simulink model "Perfect_Lineaer"  (R2017a)
settings: Solver=VariableStepAuto  StartTime=0.0  StopTime=17  FixedStep=0.01  RelTol=1e-3
values from neighbouring files (symbols this model uses):
  A = [-4.65E-06	0.0001701	-0.0002836	0	0	0	-2.56E-06	-7.97E-06	3.61E-06 ... (first row only)    [surfaces_setup_test.m]
  A0 = [-4.65E-06	0.0001701	-0.0002836	0	0	0	0	-1.43	0 ... (first row only)    [surfaces_setup_test.m]
  a0_s2345 = [0;0;0.05;0.05]    [HW5_4_surfaces.m]    (also in TEST_aerosetup.m; surfaces_setup_test.m)
  A_2345 = c_2345.*b_2345    [HW5_4_surfaces.m]    (also in TEST_aerosetup.m; surfaces_setup_test.m)
  Aileron_left = 0    [HW5_4_surfaces.m]    (also in TEST_aerosetup.m; surfaces_setup_test.m)
  Aileron_right = 0    [HW5_4_surfaces.m]    (also in TEST_aerosetup.m; surfaces_setup_test.m)
  B = [-7.98E-09	7.83E-09	1.68E-09	2.75E-10 ... (first row only)    [surfaces_setup_test.m]
  B0 = [-6.2	6.2	0	0.45 ... (first row only)    [surfaces_setup_test.m]
  c_2345 = [0.075;0.08;0.1;0.1]    [HW5_4_surfaces.m]    (also in TEST_aerosetup.m; surfaces_setup_test.m)
  CD0_s2345 = [0.01;0.01;0.01;0.01]    [HW5_4_surfaces.m]    (also in TEST_aerosetup.m; surfaces_setup_test.m)
  CDa_s2345 = [1;1;1;1]    [HW5_4_surfaces.m]    (also in TEST_aerosetup.m; surfaces_setup_test.m)
  CL0_2345 = [0;0; 0.05; 0.05]    [HW5_4_surfaces.m]    (also in TEST_aerosetup.m; surfaces_setup_test.m)
  CLa = 2*pi*(r./(2+r))    [HW5_4_surfaces.m]    (also in TEST_aerosetup.m; surfaces_setup_test.m)
  CM0_s2345 = [0;0;-0.05;-0.05]    [HW5_4_surfaces.m]    (also in TEST_aerosetup.m; surfaces_setup_test.m)
  CMa_s2345 = [0; 0; 0; 0]    [HW5_4_surfaces.m]    (also in TEST_aerosetup.m; surfaces_setup_test.m)
  e_s2345 = [0.8;0.8;0.9;0.9]    [HW5_4_surfaces.m]    (also in TEST_aerosetup.m; surfaces_setup_test.m)
  elevator = 0    [HW5_4_surfaces.m]    (also in TEST_aerosetup.m; surfaces_setup_test.m)
  Fext_N = -g_EN * m    [HW5_4_surfaces.m]    (also in TEST_aerosetup.m = [10 10 10]; surfaces_setup_test.m)
  g_EN = [0; 0; 9.81]    [HW5_4_surfaces.m]    (also in TEST_aerosetup.m = [0; 0; 9.8]; surfaces_setup_test.m)
  i_s2345 = [0; 0; 0.05; 0.05;]    [HW5_4_surfaces.m]    (also in TEST_aerosetup.m; surfaces_setup_test.m)
  J_cgp = ones(3)    [surfaces_setup_test.m]
  M_total = sum(MnG(:,1))/1000    [HW5_4_surfaces.m]    (also in TEST_aerosetup.m; surfaces_setup_test.m = sum(MnG1(:,1))/1000)
  Mext_B = [0; 0; 0]    [HW5_4_surfaces.m]    (also in TEST_aerosetup.m = [1; 1; 1]; surfaces_setup_test.m)
  p_E_BE_ini = p_E_BE_ini_deg .* [deg2rad; deg2rad; 1]    [HW5_4_surfaces.m]    (also in TEST_aerosetup.m; surfaces_setup_test.m)
  r = b_2345./c_2345    [HW5_4_surfaces.m]    (also in TEST_aerosetup.m; surfaces_setup_test.m)
  Rearth = 6371000    [HW5_4_surfaces.m]    (also in TEST_aerosetup.m; surfaces_setup_test.m)
  rudder = 0    [HW5_4_surfaces.m]    (also in TEST_aerosetup.m; surfaces_setup_test.m)
  Theta_ini = Theta_ini_deg * deg2rad    [HW5_4_surfaces.m]    (also in TEST_aerosetup.m; surfaces_setup_test.m)
  U0 = [Aileron_right;Aileron_left;elevator;rudder]    [surfaces_setup_test.m]
  v_N_AE = [0;0;0]    [HW5_4_surfaces.m]    (also in TEST_aerosetup.m; surfaces_setup_test.m)
  Vbbe_int = [10; 0; 0]    [HW5_4_surfaces.m]    (also in TEST_aerosetup.m; surfaces_setup_test.m = [5; 0; 0])
  w_B_BE_ini = [1e0; 1e-2; 1e-2]    [HW5_4_surfaces.m]    (also in TEST_aerosetup.m; surfaces_setup_test.m)
  X0 = [w_B_BE_ini;Theta_ini;Vbbe_int]    [surfaces_setup_test.m]
  xyz_s = [[-0.76 0 0.16];[-0.76 0 -0.09];[-0.23 0.44 0];[-0.23 -0.44 0];]    [HW5_4_surfaces.m]    (also in TEST_aerosetup.m; surfaces_setup_test.m)
undefined symbols (not defined in the file or in its folder): Discrete, Earth, K, Time, WGS84
libraries: simulink x83, aerolibfltsims x5, dspsrcs4 x4, simulink_extras x4, dspinverses x3, vrlib x2, sharedtransform x1, aerolibtransform2 x1, aerolibutil x1, sharedutil x1, ctrlSharedLib x1
(part 7 of 8)

== system Perfect_Lineaer/Command size/Subsystem3/selector ==
  note: Outer loop
  In1 : Inport
  Demux : Demux  Outputs=9
  Demux1 : Demux  Outputs=3
  MATLAB Function : MATLAB Function  TreatAsAtomicUnit=on
  Mux : Mux  Inputs=8
  Mux1 : Mux  Inputs=3
  Scope : Scope
  Terminator : Terminator
  Terminator1 : Terminator
  Terminator2 : Terminator
  Out1 : Outport
  Out2 : Outport  Port=2
  wires:
  Mux1/1 -> Scope/1
  Demux/9 -> Mux/8
  Demux/8 -> Out1/1
  Mux/1 -> Terminator/1
  Demux/7 -> Mux/7
  Demux/6 -> Mux/6, Mux1/3
  Demux/4 -> MATLAB Function/1(phi), Mux/4, Mux1/1
  In1/1 -> Demux/1
  Demux/2 -> MATLAB Function/5(R), Mux/2
  Demux/3 -> Mux/3
  Demux/1 -> MATLAB Function/4(Q), MATLAB Function/3(P), Mux/1
  Demux/5 -> MATLAB Function/2(theta), Mux/5, Mux1/2
  MATLAB Function/1(euler_dot) -> Demux1/1
  Demux1/2 -> Out2/1
  Demux1/1 -> Terminator1/1
  Demux1/3 -> Terminator2/1

== system Perfect_Lineaer/Command size/Subsystem4/selector ==
  note: Outer loop
  In1 : Inport
  Demux : Demux  Outputs=9
  Demux1 : Demux  Outputs=3
  MATLAB Function : MATLAB Function  TreatAsAtomicUnit=on
  Mux : Mux  Inputs=8
  Mux1 : Mux  Inputs=3
  Scope : Scope
  Terminator : Terminator
  Terminator1 : Terminator
  Terminator2 : Terminator
  Out1 : Outport
  Out2 : Outport  Port=2
  wires:
  Demux1/2 -> Terminator1/1
  Demux/7 -> Mux/7
  Demux/3 -> Mux/3
  Mux/1 -> Terminator/1
  Demux/2 -> MATLAB Function/5(R), Mux/2
  In1/1 -> Demux/1
  Demux/5 -> MATLAB Function/2(theta), Mux/5, Mux1/2
  Demux/9 -> Mux/8
  Demux/6 -> Mux/6, Mux1/3
  Demux1/3 -> Terminator2/1
  MATLAB Function/1(euler_dot) -> Demux1/1
  Mux1/1 -> Scope/1
  Demux/4 -> MATLAB Function/1(phi), Mux/4, Mux1/1
  Demux/1 -> MATLAB Function/4(Q), MATLAB Function/3(P), Mux/1
  Demux1/1 -> Out2/1
  Demux/8 -> Out1/1

== system Perfect_Lineaer/Command size/Subsystem9/selector ==
  note: Outer loop
  In1 : Inport
  Demux : Demux  Outputs=9
  Demux1 : Demux  Outputs=3
  MATLAB Function : MATLAB Function  TreatAsAtomicUnit=on
  Mux : Mux  Inputs=8
  Mux1 : Mux  Inputs=3
  Scope : Scope
  Terminator : Terminator
  Terminator1 : Terminator
  Terminator2 : Terminator
  Out1 : Outport
  Out2 : Outport  Port=2
  wires:
  Demux1/2 -> Terminator1/1
  Demux/7 -> Mux/7
  Demux/3 -> Mux/3
  Mux/1 -> Terminator/1
  Demux/2 -> MATLAB Function/5(R), Mux/2
  In1/1 -> Demux/1
  Demux/5 -> MATLAB Function/2(theta), Mux/5, Mux1/2
  Demux/9 -> Mux/8
  Demux/6 -> Mux/6, Mux1/3
  Demux1/3 -> Terminator2/1
  MATLAB Function/1(euler_dot) -> Demux1/1
  Mux1/1 -> Scope/1
  Demux/4 -> MATLAB Function/1(phi), Mux/4, Mux1/1
  Demux/1 -> MATLAB Function/4(Q), MATLAB Function/3(P), Mux/1
  Demux1/1 -> Out2/1
  Demux/8 -> Out1/1

== system Perfect_Lineaer/Decoupled/Subsystem/selector ==
  note: Outer loop
  In1 : Inport
  Demux : Demux  Outputs=9
  Demux1 : Demux  Outputs=3
  MATLAB Function : MATLAB Function  TreatAsAtomicUnit=on
  Mux : Mux  Inputs=8
  Mux1 : Mux  Inputs=3
  Scope : Scope
  Terminator : Terminator
  Terminator1 : Terminator
  Terminator2 : Terminator
  Out1 : Outport
  Out2 : Outport  Port=2
  wires:
  MATLAB Function/1(euler_dot) -> Demux1/1
  Demux1/1 -> Terminator1/1
  In1/1 -> Demux/1
  Demux/9 -> Mux/8
  Demux/5 -> MATLAB Function/2(theta), Mux/5, Mux1/2
  Demux/2 -> MATLAB Function/5(R), Mux/2
  Demux/6 -> Mux/6, Mux1/3
  Demux/1 -> MATLAB Function/4(Q), MATLAB Function/3(P), Mux/1
  Demux/3 -> Mux/3
  Mux/1 -> Terminator/1
  Demux/7 -> Mux/7
  Demux/4 -> MATLAB Function/1(phi), Mux/4, Mux1/1
  Demux/8 -> Out1/1
  Mux1/1 -> Scope/1
  Demux1/3 -> Out2/1
  Demux1/2 -> Terminator2/1

== system Perfect_Lineaer/Decoupled/Subsystem1/selector ==
  note: Outer loop
  In1 : Inport
  Demux : Demux  Outputs=9
  Demux1 : Demux  Outputs=3
  MATLAB Function : MATLAB Function  TreatAsAtomicUnit=on
  Mux : Mux  Inputs=8
  Mux1 : Mux  Inputs=3
  Scope : Scope
  Terminator : Terminator
  Terminator1 : Terminator
  Terminator2 : Terminator
  Out1 : Outport
  Out2 : Outport  Port=2
  wires:
  Mux1/1 -> Scope/1
  Demux/9 -> Mux/8
  Demux/8 -> Out1/1
  Mux/1 -> Terminator/1
  Demux/7 -> Mux/7
  Demux/6 -> Mux/6, Mux1/3
  Demux/4 -> MATLAB Function/1(phi), Mux/4, Mux1/1
  In1/1 -> Demux/1
  Demux/2 -> MATLAB Function/5(R), Mux/2
  Demux/3 -> Mux/3
  Demux/1 -> MATLAB Function/4(Q), MATLAB Function/3(P), Mux/1
  Demux/5 -> MATLAB Function/2(theta), Mux/5, Mux1/2
  MATLAB Function/1(euler_dot) -> Demux1/1
  Demux1/2 -> Out2/1
  Demux1/1 -> Terminator1/1
  Demux1/3 -> Terminator2/1

== system Perfect_Lineaer/Decoupled/Subsystem5/selector ==
  note: Outer loop
  In1 : Inport
  Demux : Demux  Outputs=9
  Demux1 : Demux  Outputs=3
  MATLAB Function : MATLAB Function  TreatAsAtomicUnit=on
  Mux : Mux  Inputs=8
  Mux1 : Mux  Inputs=3
  Scope : Scope
  Terminator : Terminator
  Terminator1 : Terminator
  Out1 : Outport
  Out2 : Outport  Port=2
  Out3 : Outport  Port=3
  wires:
  MATLAB Function/1(euler_dot) -> Demux1/1
  Demux1/1 -> Terminator1/1
  In1/1 -> Demux/1
  Demux/9 -> Mux/8
  Demux/5 -> MATLAB Function/2(theta), Mux/5, Mux1/2
  Demux/2 -> MATLAB Function/5(R), Mux/2
  Demux/6 -> Mux/6, Mux1/3
  Demux/1 -> MATLAB Function/4(Q), MATLAB Function/3(P), Mux/1
  Demux/3 -> Mux/3
  Mux/1 -> Terminator/1
  Demux/7 -> Mux/7
  Demux/4 -> MATLAB Function/1(phi), Mux/4, Mux1/1
  Demux1/2 -> Out2/1
  Demux/8 -> Out1/1
  Mux1/1 -> Scope/1
  Demux1/3 -> Out3/1

== system Perfect_Lineaer/Decoupled/Subsystem9/selector ==
  note: Outer loop
  In1 : Inport
  Demux : Demux  Outputs=9
  Demux1 : Demux  Outputs=3
  MATLAB Function : MATLAB Function  TreatAsAtomicUnit=on
  Mux : Mux  Inputs=8
  Mux1 : Mux  Inputs=3
  Scope : Scope
  Terminator : Terminator
  Terminator1 : Terminator
  Terminator2 : Terminator
  Out1 : Outport
  Out2 : Outport  Port=2
  wires:
  Demux1/2 -> Terminator1/1
  Demux/7 -> Mux/7
  Demux/3 -> Mux/3
  Mux/1 -> Terminator/1
  Demux/2 -> MATLAB Function/5(R), Mux/2
  In1/1 -> Demux/1
  Demux/5 -> MATLAB Function/2(theta), Mux/5, Mux1/2
  Demux/9 -> Mux/8
  Demux/6 -> Mux/6, Mux1/3
  Demux1/3 -> Terminator2/1
  MATLAB Function/1(euler_dot) -> Demux1/1
  Mux1/1 -> Scope/1
  Demux/4 -> MATLAB Function/1(phi), Mux/4, Mux1/1
  Demux/1 -> MATLAB Function/4(Q), MATLAB Function/3(P), Mux/1
  Demux1/1 -> Out2/1
  Demux/8 -> Out1/1

== system Perfect_Lineaer/Pilot command(STT)/Subsystem/selector ==
  note: Outer loop
  In1 : Inport
  Demux : Demux  Outputs=9
  Demux1 : Demux  Outputs=3
  MATLAB Function : MATLAB Function  TreatAsAtomicUnit=on
  Mux : Mux  Inputs=8
  Mux1 : Mux  Inputs=3
  Scope : Scope
  Terminator : Terminator
  Terminator1 : Terminator
  Terminator2 : Terminator
  Out1 : Outport
  Out2 : Outport  Port=2
  wires:
  MATLAB Function/1(euler_dot) -> Demux1/1
  Demux1/1 -> Terminator1/1
  In1/1 -> Demux/1
  Demux/9 -> Mux/8
  Demux/5 -> MATLAB Function/2(theta), Mux/5, Mux1/2
  Demux/2 -> MATLAB Function/5(R), Mux/2
  Demux/6 -> Mux/6, Mux1/3
  Demux/1 -> MATLAB Function/4(Q), MATLAB Function/3(P), Mux/1
  Demux/3 -> Mux/3
  Mux/1 -> Terminator/1
  Demux/7 -> Mux/7
  Demux/4 -> MATLAB Function/1(phi), Mux/4, Mux1/1
  Demux/8 -> Out1/1
  Mux1/1 -> Scope/1
  Demux1/3 -> Out2/1
  Demux1/2 -> Terminator2/1

== system Perfect_Lineaer/Pilot command(STT)/Subsystem1/selector ==
  note: Outer loop
  In1 : Inport
  Demux : Demux  Outputs=9
  Demux1 : Demux  Outputs=3
  MATLAB Function : MATLAB Function  TreatAsAtomicUnit=on
  Mux : Mux  Inputs=8
  Mux1 : Mux  Inputs=3
  Scope : Scope
  Terminator : Terminator
  Terminator1 : Terminator
  Terminator2 : Terminator
  Out1 : Outport
  Out2 : Outport  Port=2
  wires:
  Mux1/1 -> Scope/1
  Demux/9 -> Mux/8
  Demux/8 -> Out1/1
  Mux/1 -> Terminator/1
  Demux/7 -> Mux/7
  Demux/6 -> Mux/6, Mux1/3
  Demux/4 -> MATLAB Function/1(phi), Mux/4, Mux1/1
  In1/1 -> Demux/1
  Demux/2 -> MATLAB Function/5(R), Mux/2
  Demux/3 -> Mux/3
  Demux/1 -> MATLAB Function/4(Q), MATLAB Function/3(P), Mux/1
  Demux/5 -> MATLAB Function/2(theta), Mux/5, Mux1/2
  MATLAB Function/1(euler_dot) -> Demux1/1
  Demux1/2 -> Out2/1
  Demux1/1 -> Terminator1/1
  Demux1/3 -> Terminator2/1

== system Perfect_Lineaer/Pilot command(STT)/Subsystem5/selector ==
  note: Outer loop
  In1 : Inport
  Demux : Demux  Outputs=9
  Demux1 : Demux  Outputs=3
  MATLAB Function : MATLAB Function  TreatAsAtomicUnit=on
  Mux : Mux  Inputs=8
  Mux1 : Mux  Inputs=3
  Scope : Scope
  Terminator : Terminator
  Terminator1 : Terminator
  Out1 : Outport
  Out2 : Outport  Port=2
  Out3 : Outport  Port=3
  wires:
  MATLAB Function/1(euler_dot) -> Demux1/1
  Demux1/1 -> Terminator1/1
  In1/1 -> Demux/1
  Demux/9 -> Mux/8
  Demux/5 -> MATLAB Function/2(theta), Mux/5, Mux1/2
  Demux/2 -> MATLAB Function/5(R), Mux/2
  Demux/6 -> Mux/6, Mux1/3
  Demux/1 -> MATLAB Function/4(Q), MATLAB Function/3(P), Mux/1
  Demux/3 -> Mux/3
  Mux/1 -> Terminator/1
  Demux/7 -> Mux/7
  Demux/4 -> MATLAB Function/1(phi), Mux/4, Mux1/1
  Demux1/2 -> Out2/1
  Demux/8 -> Out1/1
  Mux1/1 -> Scope/1
  Demux1/3 -> Out3/1

== system Perfect_Lineaer/Really skid to turn/Subsystem5/selector ==
  note: Outer loop
  In1 : Inport
  Demux : Demux  Outputs=9
  Demux1 : Demux  Outputs=3
  MATLAB Function : MATLAB Function  TreatAsAtomicUnit=on
  Mux : Mux  Inputs=8
  Mux1 : Mux  Inputs=3
  Scope : Scope
  Terminator : Terminator
  Terminator1 : Terminator
  Out1 : Outport
  Out2 : Outport  Port=2
  Out3 : Outport  Port=3
  wires:
  MATLAB Function/1(euler_dot) -> Demux1/1
  Demux1/1 -> Terminator1/1
  In1/1 -> Demux/1
  Demux/9 -> Mux/8
  Demux/5 -> MATLAB Function/2(theta), Mux/5, Mux1/2
  Demux/2 -> MATLAB Function/5(R), Mux/2
  Demux/6 -> Mux/6, Mux1/3
  Demux/1 -> MATLAB Function/4(Q), MATLAB Function/3(P), Mux/1
  Demux/3 -> Mux/3
  Mux/1 -> Terminator/1
  Demux/7 -> Mux/7
  Demux/4 -> MATLAB Function/1(phi), Mux/4, Mux1/1
  Demux1/2 -> Out2/1
  Demux/8 -> Out1/1
  Mux1/1 -> Scope/1
  Demux1/3 -> Out3/1

== system Perfect_Lineaer/Really skid to turn/Subsystem8/selector ==
  note: Outer loop
  In1 : Inport
  Demux : Demux  Outputs=9
  Demux1 : Demux  Outputs=3
  MATLAB Function : MATLAB Function  TreatAsAtomicUnit=on
  Mux : Mux  Inputs=8
  Mux1 : Mux  Inputs=3
  Scope : Scope
  Terminator : Terminator
  Terminator1 : Terminator
  Terminator2 : Terminator
  Out1 : Outport
  Out2 : Outport  Port=2
  wires:
  Demux1/2 -> Terminator1/1
  Demux/7 -> Mux/7
  Demux/3 -> Mux/3
  Mux/1 -> Terminator/1
  Demux/2 -> MATLAB Function/5(R), Mux/2
  In1/1 -> Demux/1
  Demux/5 -> MATLAB Function/2(theta), Mux/5, Mux1/2
  Demux/9 -> Mux/8
  Demux/6 -> Mux/6, Mux1/3
  Demux1/3 -> Terminator2/1
  MATLAB Function/1(euler_dot) -> Demux1/1
  Mux1/1 -> Scope/1
  Demux/4 -> MATLAB Function/1(phi), Mux/4, Mux1/1
  Demux/1 -> MATLAB Function/4(Q), MATLAB Function/3(P), Mux/1
  Demux1/1 -> Out2/1
  Demux/8 -> Out1/1

== system Perfect_Lineaer/Really skid to turn/Subsystem9/selector ==
  note: Outer loop
  In1 : Inport
  Demux : Demux  Outputs=9
  Demux1 : Demux  Outputs=3
  MATLAB Function : MATLAB Function  TreatAsAtomicUnit=on
  Mux : Mux  Inputs=8
  Mux1 : Mux  Inputs=3
  Scope : Scope
  Terminator : Terminator
  Terminator1 : Terminator
  Terminator2 : Terminator
  Out1 : Outport
  Out2 : Outport  Port=2
  wires:
  Demux1/2 -> Terminator1/1
  Demux/7 -> Mux/7
  Demux/3 -> Mux/3
  Mux/1 -> Terminator/1
  Demux/2 -> MATLAB Function/5(R), Mux/2
  In1/1 -> Demux/1
  Demux/5 -> MATLAB Function/2(theta), Mux/5, Mux1/2
  Demux/9 -> Mux/8
  Demux/6 -> Mux/6, Mux1/3
  Demux1/3 -> Terminator2/1
  MATLAB Function/1(euler_dot) -> Demux1/1
  Mux1/1 -> Scope/1
  Demux/4 -> MATLAB Function/1(phi), Mux/4, Mux1/1
  Demux/1 -> MATLAB Function/4(Q), MATLAB Function/3(P), Mux/1
  Demux1/1 -> Out2/1
  Demux/8 -> Out1/1

== system Perfect_Lineaer/Skid to turn (Lateral Dynamics don't change!)/Subsystem/selector ==
  note: Outer loop
  In1 : Inport
  Demux : Demux  Outputs=9
  Mux : Mux  Inputs=8
  Mux1 : Mux  Inputs=3
  Scope : Scope
  Terminator : Terminator
  Out1 : Outport
  Out2 : Outport  Port=2
  wires:
  Demux/5 -> Mux1/2, Mux/5
  Demux/1 -> Mux/1
  Demux/3 -> Out2/1, Mux/3
  Demux/2 -> Mux/2
  In1/1 -> Demux/1
  Demux/4 -> Mux1/1, Mux/4
  Demux/6 -> Mux1/3, Mux/6
  Demux/7 -> Mux/7
  Mux/1 -> Terminator/1
  Demux/8 -> Out1/1
  Demux/9 -> Mux/8
  Mux1/1 -> Scope/1

== system Perfect_Lineaer/Skid to turn (Lateral Dynamics don't change!)/Subsystem1/selector ==
  note: Outer loop
  In1 : Inport
  Demux : Demux  Outputs=9
  Mux : Mux  Inputs=8
  Mux1 : Mux  Inputs=3
  Scope : Scope
  Terminator : Terminator
  Out1 : Outport
  Out2 : Outport  Port=2
  wires:
  Demux/5 -> Mux1/2, Mux/5
  Demux/1 -> Mux/1
  Demux/3 -> Mux/3
  Demux/2 -> Out2/1, Mux/2
  In1/1 -> Demux/1
  Demux/4 -> Mux1/1, Mux/4
  Demux/6 -> Mux1/3, Mux/6
  Demux/7 -> Mux/7
  Mux/1 -> Terminator/1
  Demux/8 -> Out1/1
  Demux/9 -> Mux/8
  Mux1/1 -> Scope/1

== system Perfect_Lineaer/Skid to turn (Lateral Dynamics don't change!)/Subsystem2/selector ==
  note: Outer loop
  In1 : Inport
  Demux : Demux  Outputs=9
  Mux : Mux  Inputs=8
  Mux1 : Mux  Inputs=3
  Scope : Scope
  Terminator : Terminator
  Out1 : Outport
  Out2 : Outport  Port=2
  wires:
  Demux/5 -> Mux1/2, Mux/5
  Demux/1 -> Mux/1
  Demux/3 -> Out2/1, Mux/3
  Demux/2 -> Mux/2
  In1/1 -> Demux/1
  Demux/4 -> Mux1/1, Mux/4
  Demux/6 -> Mux1/3, Mux/6
  Demux/7 -> Mux/7
  Mux/1 -> Terminator/1
  Demux/8 -> Out1/1
  Demux/9 -> Mux/8
  Mux1/1 -> Scope/1

== system Perfect_Lineaer/Skid to turn (Lateral Dynamics don't change!)/Subsystem3/selector ==
  note: Outer loop
  In1 : Inport
  Demux : Demux  Outputs=9
  Mux : Mux  Inputs=8
  Mux1 : Mux  Inputs=3
  Scope : Scope
  Terminator : Terminator
  Out1 : Outport
  Out2 : Outport  Port=2
  wires:
  Demux/5 -> Mux1/2, Mux/5
  Demux/1 -> Mux/1
  Demux/3 -> Out2/1, Mux/3
  Demux/2 -> Mux/2
  In1/1 -> Demux/1
  Demux/4 -> Mux1/1, Mux/4
  Demux/6 -> Mux1/3, Mux/6
  Demux/7 -> Mux/7
  Mux/1 -> Terminator/1
  Demux/8 -> Out1/1
  Demux/9 -> Mux/8
  Mux1/1 -> Scope/1

== system Perfect_Lineaer/Skid to turn (Lateral Dynamics don't change!)/Subsystem4/selector ==
  note: Outer loop
  In1 : Inport
  Demux : Demux  Outputs=9
  Mux : Mux  Inputs=8
  Mux1 : Mux  Inputs=3
  Scope : Scope
  Terminator : Terminator
  Out1 : Outport
  Out2 : Outport  Port=2
  wires:
  Demux/5 -> Mux1/2, Mux/5
  Demux/1 -> Mux/1
  Demux/3 -> Out2/1, Mux/3
  Demux/2 -> Mux/2
  In1/1 -> Demux/1
  Demux/4 -> Mux1/1, Mux/4
  Demux/6 -> Mux1/3, Mux/6
  Demux/7 -> Mux/7
  Mux/1 -> Terminator/1
  Demux/8 -> Out1/1
  Demux/9 -> Mux/8
  Mux1/1 -> Scope/1

== system Perfect_Lineaer/Skid to turn (Lateral Dynamics don't change!)/Subsystem5/selector ==
  note: Outer loop
  In1 : Inport
  Demux : Demux  Outputs=9
  Mux : Mux  Inputs=8
  Mux1 : Mux  Inputs=3
  Scope : Scope
  Terminator : Terminator
  Out1 : Outport
  yaw : Outport  Port=2
  pitch : Outport  Port=3
  wires:
  Demux/5 -> Mux1/2, Mux/5
  Demux/1 -> Mux/1
  Demux/3 -> yaw/1, Mux/3
  Demux/2 -> pitch/1, Mux/2
  In1/1 -> Demux/1
  Demux/4 -> Mux1/1, Mux/4
  Demux/6 -> Mux1/3, Mux/6
  Demux/7 -> Mux/7
  Mux/1 -> Terminator/1
  Demux/8 -> Out1/1
  Demux/9 -> Mux/8
  Mux1/1 -> Scope/1

== system Perfect_Lineaer/Skid to turn (Lateral Dynamics don't change!)/Subsystem6/selector ==
  note: Outer loop
  In1 : Inport
  Demux : Demux  Outputs=9
  Mux : Mux  Inputs=8
  Mux1 : Mux  Inputs=3
  Scope : Scope
  Terminator : Terminator
  Out1 : Outport
  Out2 : Outport  Port=2
  wires:
  Demux/5 -> Mux1/2, Mux/5
  Demux/1 -> Mux/1
  Demux/3 -> Out2/1, Mux/3
  Demux/2 -> Mux/2
  In1/1 -> Demux/1
  Demux/4 -> Mux1/1, Mux/4
  Demux/6 -> Mux1/3, Mux/6
  Demux/7 -> Mux/7
  Mux/1 -> Terminator/1
  Demux/8 -> Out1/1
  Demux/9 -> Mux/8
  Mux1/1 -> Scope/1

== system Perfect_Lineaer/Skid to turn (Lateral Dynamics don't change!)/Subsystem7/selector ==
  note: Outer loop
  In1 : Inport
  Demux : Demux  Outputs=9
  Mux : Mux  Inputs=8
  Mux1 : Mux  Inputs=3
  Scope : Scope
  Terminator : Terminator
  Out1 : Outport
  Out2 : Outport  Port=2
  wires:
  Demux/5 -> Mux1/2, Mux/5
  Demux/1 -> Out2/1, Mux/1
  Demux/3 -> Mux/3
  Demux/2 -> Mux/2
  In1/1 -> Demux/1
  Demux/4 -> Mux1/1, Mux/4
  Demux/6 -> Mux1/3, Mux/6
  Demux/7 -> Mux/7
  Mux/1 -> Terminator/1
  Demux/8 -> Out1/1
  Demux/9 -> Mux/8
  Mux1/1 -> Scope/1

== system Perfect_Lineaer/Skid to turn (Lateral Dynamics don't change!)/Subsystem8/selector ==
  note: Outer loop
  In1 : Inport
  Demux : Demux  Outputs=9
  Mux : Mux  Inputs=8
  Mux1 : Mux  Inputs=3
  Scope : Scope
  Terminator : Terminator
  Out1 : Outport
  Out2 : Outport  Port=2
  wires:
  Demux/5 -> Mux1/2, Mux/5
  Demux/1 -> Out2/1, Mux/1
  Demux/3 -> Mux/3
  Demux/2 -> Mux/2
  In1/1 -> Demux/1
  Demux/4 -> Mux1/1, Mux/4
  Demux/6 -> Mux1/3, Mux/6
  Demux/7 -> Mux/7
  Mux/1 -> Terminator/1
  Demux/8 -> Out1/1
  Demux/9 -> Mux/8
  Mux1/1 -> Scope/1

== system Perfect_Lineaer/Skid to turn (Lateral Dynamics don't change!)/Subsystem9/selector ==
  note: Outer loop
  In1 : Inport
  Demux : Demux  Outputs=9
  Mux : Mux  Inputs=8
  Mux1 : Mux  Inputs=3
  Scope : Scope
  Terminator : Terminator
  Out1 : Outport
  Out2 : Outport  Port=2
  wires:
  Demux/5 -> Mux1/2, Mux/5
  Demux/1 -> Out2/1, Mux/1
  Demux/3 -> Mux/3
  Demux/2 -> Mux/2
  In1/1 -> Demux/1
  Demux/4 -> Mux1/1, Mux/4
  Demux/6 -> Mux1/3, Mux/6
  Demux/7 -> Mux/7
  Mux/1 -> Terminator/1
  Demux/8 -> Out1/1
  Demux/9 -> Mux/8
  Mux1/1 -> Scope/1

== system Perfect_Lineaer/Skid to turn (Lateral Dynamics)1/Subsystem/selector ==
  note: Outer loop
  In1 : Inport
  Demux : Demux  Outputs=9
  Mux : Mux  Inputs=8
  Mux1 : Mux  Inputs=3
  Scope : Scope
  Terminator : Terminator
  Out1 : Outport
  Out2 : Outport  Port=2
  wires:
  Demux/5 -> Mux1/2, Mux/5
  Demux/1 -> Mux/1
  Demux/3 -> Out2/1, Mux/3
  Demux/2 -> Mux/2
  In1/1 -> Demux/1
  Demux/4 -> Mux1/1, Mux/4
  Demux/6 -> Mux1/3, Mux/6
  Demux/7 -> Mux/7
  Mux/1 -> Terminator/1
  Demux/8 -> Out1/1
  Demux/9 -> Mux/8
  Mux1/1 -> Scope/1

== system Perfect_Lineaer/Skid to turn (Lateral Dynamics)1/Subsystem1/selector ==
  note: Outer loop
  In1 : Inport
  Demux : Demux  Outputs=9
  Mux : Mux  Inputs=8
  Mux1 : Mux  Inputs=3
  Scope : Scope
  Terminator : Terminator
  Out1 : Outport
  Out2 : Outport  Port=2
  wires:
  Demux/5 -> Mux1/2, Mux/5
  Demux/1 -> Mux/1
  Demux/3 -> Mux/3
  Demux/2 -> Out2/1, Mux/2
  In1/1 -> Demux/1
  Demux/4 -> Mux1/1, Mux/4
  Demux/6 -> Mux1/3, Mux/6
  Demux/7 -> Mux/7
  Mux/1 -> Terminator/1
  Demux/8 -> Out1/1
  Demux/9 -> Mux/8
  Mux1/1 -> Scope/1

== system Perfect_Lineaer/Skid to turn (Lateral Dynamics)1/Subsystem2/selector ==
  note: Outer loop
  In1 : Inport
  Demux : Demux  Outputs=9
  Mux : Mux  Inputs=8
  Mux1 : Mux  Inputs=3
  Scope : Scope
  Terminator : Terminator
  Out1 : Outport
  Out2 : Outport  Port=2
  wires:
  Demux/5 -> Mux1/2, Mux/5
  Demux/1 -> Mux/1
  Demux/3 -> Out2/1, Mux/3
  Demux/2 -> Mux/2
  In1/1 -> Demux/1
  Demux/4 -> Mux1/1, Mux/4
  Demux/6 -> Mux1/3, Mux/6
  Demux/7 -> Mux/7
  Mux/1 -> Terminator/1
  Demux/8 -> Out1/1
  Demux/9 -> Mux/8
  Mux1/1 -> Scope/1

== system Perfect_Lineaer/Skid to turn (Lateral Dynamics)1/Subsystem3/selector ==
  note: Outer loop
  In1 : Inport
  Demux : Demux  Outputs=9
  Mux : Mux  Inputs=8
  Mux1 : Mux  Inputs=3
  Scope : Scope
  Terminator : Terminator
  Out1 : Outport
  Out2 : Outport  Port=2
  wires:
  Demux/5 -> Mux1/2, Mux/5
  Demux/1 -> Mux/1
  Demux/3 -> Out2/1, Mux/3
  Demux/2 -> Mux/2
  In1/1 -> Demux/1
  Demux/4 -> Mux1/1, Mux/4
  Demux/6 -> Mux1/3, Mux/6
  Demux/7 -> Mux/7
  Mux/1 -> Terminator/1
  Demux/8 -> Out1/1
  Demux/9 -> Mux/8
  Mux1/1 -> Scope/1

== system Perfect_Lineaer/Skid to turn (Lateral Dynamics)1/Subsystem4/selector ==
  note: Outer loop
  In1 : Inport
  Demux : Demux  Outputs=9
  Mux : Mux  Inputs=8
  Mux1 : Mux  Inputs=3
  Scope : Scope
  Terminator : Terminator
  Out1 : Outport
  Out2 : Outport  Port=2
  wires:
  Demux/5 -> Mux1/2, Mux/5
  Demux/1 -> Mux/1
  Demux/3 -> Out2/1, Mux/3
  Demux/2 -> Mux/2
  In1/1 -> Demux/1
  Demux/4 -> Mux1/1, Mux/4
  Demux/6 -> Mux1/3, Mux/6
  Demux/7 -> Mux/7
  Mux/1 -> Terminator/1
  Demux/8 -> Out1/1
  Demux/9 -> Mux/8
  Mux1/1 -> Scope/1

== system Perfect_Lineaer/Skid to turn (Lateral Dynamics)1/Subsystem5/selector ==
  note: Outer loop
  In1 : Inport
  Demux : Demux  Outputs=9
  Mux : Mux  Inputs=8
  Mux1 : Mux  Inputs=3
  Scope : Scope
  Terminator : Terminator
  Out1 : Outport
  yaw : Outport  Port=2
  pitch : Outport  Port=3
  wires:
  Demux/5 -> Mux1/2, Mux/5
  Demux/1 -> Mux/1
  Demux/3 -> yaw/1, Mux/3
  Demux/2 -> pitch/1, Mux/2
  In1/1 -> Demux/1
  Demux/4 -> Mux1/1, Mux/4
  Demux/6 -> Mux1/3, Mux/6
  Demux/7 -> Mux/7
  Mux/1 -> Terminator/1
  Demux/8 -> Out1/1
  Demux/9 -> Mux/8
  Mux1/1 -> Scope/1

== system Perfect_Lineaer/Skid to turn (Lateral Dynamics)1/Subsystem6/selector ==
  note: Outer loop
  In1 : Inport
  Demux : Demux  Outputs=9
  Mux : Mux  Inputs=8
  Mux1 : Mux  Inputs=3
  Scope : Scope
  Terminator : Terminator
  Out1 : Outport
  Out2 : Outport  Port=2
  wires:
  Demux/5 -> Mux1/2, Mux/5
  Demux/1 -> Mux/1
  Demux/3 -> Out2/1, Mux/3
  Demux/2 -> Mux/2
  In1/1 -> Demux/1
  Demux/4 -> Mux1/1, Mux/4
  Demux/6 -> Mux1/3, Mux/6
  Demux/7 -> Mux/7
  Mux/1 -> Terminator/1
  Demux/8 -> Out1/1
  Demux/9 -> Mux/8
  Mux1/1 -> Scope/1

== system Perfect_Lineaer/Skid to turn (Lateral Dynamics)1/Subsystem7/selector ==
  note: Outer loop
  In1 : Inport
  Demux : Demux  Outputs=9
  Mux : Mux  Inputs=8
  Mux1 : Mux  Inputs=3
  Scope : Scope
  Terminator : Terminator
  Out1 : Outport
  Out2 : Outport  Port=2
  wires:
  Demux/5 -> Mux1/2, Mux/5
  Demux/1 -> Out2/1, Mux/1
  Demux/3 -> Mux/3
  Demux/2 -> Mux/2
  In1/1 -> Demux/1
  Demux/4 -> Mux1/1, Mux/4
  Demux/6 -> Mux1/3, Mux/6
  Demux/7 -> Mux/7
  Mux/1 -> Terminator/1
  Demux/8 -> Out1/1
  Demux/9 -> Mux/8
  Mux1/1 -> Scope/1

== system Perfect_Lineaer/Skid to turn (Lateral Dynamics)1/Subsystem8/selector ==
  note: Outer loop
  In1 : Inport
  Demux : Demux  Outputs=9
  Mux : Mux  Inputs=8
  Mux1 : Mux  Inputs=3
  Scope : Scope
  Terminator : Terminator
  Out1 : Outport
  Out2 : Outport  Port=2
  wires:
  Demux/5 -> Mux1/2, Mux/5
  Demux/1 -> Out2/1, Mux/1
  Demux/3 -> Mux/3
  Demux/2 -> Mux/2
  In1/1 -> Demux/1
  Demux/4 -> Mux1/1, Mux/4
  Demux/6 -> Mux1/3, Mux/6
  Demux/7 -> Mux/7
  Mux/1 -> Terminator/1
  Demux/8 -> Out1/1
  Demux/9 -> Mux/8
  Mux1/1 -> Scope/1

== system Perfect_Lineaer/Skid to turn (Lateral Dynamics)1/Subsystem9/selector ==
  note: Outer loop
  In1 : Inport
  Demux : Demux  Outputs=9
  Mux : Mux  Inputs=8
  Mux1 : Mux  Inputs=3
  Scope : Scope
  Terminator : Terminator
  Out1 : Outport
  Out2 : Outport  Port=2
  wires:
  Demux/5 -> Mux1/2, Mux/5
  Demux/1 -> Out2/1, Mux/1
  Demux/3 -> Mux/3
  Demux/2 -> Mux/2
  In1/1 -> Demux/1
  Demux/4 -> Mux1/1, Mux/4
  Demux/6 -> Mux1/3, Mux/6
  Demux/7 -> Mux/7
  Mux/1 -> Terminator/1
  Demux/8 -> Out1/1
  Demux/9 -> Mux/8
  Mux1/1 -> Scope/1

== system Perfect_Lineaer/Skid to turn (Lateral Dynamics)2/Subsystem/selector ==
  note: Outer loop
  In1 : Inport
  Demux : Demux  Outputs=9
  Demux1 : Demux  Outputs=3
  MATLAB Function : MATLAB Function  TreatAsAtomicUnit=on
  Mux : Mux  Inputs=8
  Mux1 : Mux  Inputs=3
  Scope : Scope
  Terminator : Terminator
  Terminator1 : Terminator
  Terminator2 : Terminator
  Out1 : Outport
  Out2 : Outport  Port=2
  wires:
  MATLAB Function/1(euler_dot) -> Demux1/1
  Demux1/1 -> Terminator1/1
  In1/1 -> Demux/1
  Demux/9 -> Mux/8
  Demux/5 -> MATLAB Function/2(theta), Mux/5, Mux1/2
  Demux/2 -> MATLAB Function/5(R), Mux/2
  Demux/6 -> Mux/6, Mux1/3
  Demux/1 -> MATLAB Function/4(Q), MATLAB Function/3(P), Mux/1
  Demux/3 -> Mux/3
  Mux/1 -> Terminator/1
  Demux/7 -> Mux/7
  Demux/4 -> MATLAB Function/1(phi), Mux/4, Mux1/1
  Demux/8 -> Out1/1
  Mux1/1 -> Scope/1
  Demux1/3 -> Out2/1
  Demux1/2 -> Terminator2/1

== system Perfect_Lineaer/Skid to turn (Lateral Dynamics)2/Subsystem1/selector ==
  note: Outer loop
  In1 : Inport
  Demux : Demux  Outputs=9
  Demux1 : Demux  Outputs=3
  MATLAB Function : MATLAB Function  TreatAsAtomicUnit=on
  Mux : Mux  Inputs=8
  Mux1 : Mux  Inputs=3
  Scope : Scope
  Terminator : Terminator
  Terminator1 : Terminator
  Terminator2 : Terminator
  Out1 : Outport
  Out2 : Outport  Port=2
  wires:
  Mux1/1 -> Scope/1
  Demux/9 -> Mux/8
  Demux/8 -> Out1/1
  Mux/1 -> Terminator/1
  Demux/7 -> Mux/7
  Demux/6 -> Mux/6, Mux1/3
  Demux/4 -> MATLAB Function/1(phi), Mux/4, Mux1/1
  In1/1 -> Demux/1
  Demux/2 -> MATLAB Function/5(R), Mux/2
  Demux/3 -> Mux/3
  Demux/1 -> MATLAB Function/4(Q), MATLAB Function/3(P), Mux/1
  Demux/5 -> MATLAB Function/2(theta), Mux/5, Mux1/2
  MATLAB Function/1(euler_dot) -> Demux1/1
  Demux1/2 -> Out2/1
  Demux1/1 -> Terminator1/1
  Demux1/3 -> Terminator2/1

== system Perfect_Lineaer/Skid to turn (Lateral Dynamics)2/Subsystem2/selector ==
  note: Outer loop
  In1 : Inport
  Demux : Demux  Outputs=9
  Mux : Mux  Inputs=8
  Mux1 : Mux  Inputs=3
  Scope : Scope
  Terminator : Terminator
  Out1 : Outport
  Out2 : Outport  Port=2
  wires:
  Mux1/1 -> Scope/1
  Demux/9 -> Mux/8
  Demux/8 -> Out1/1
  Mux/1 -> Terminator/1
  Demux/7 -> Mux/7
  Demux/6 -> Mux/6, Mux1/3
  Demux/4 -> Mux/4, Mux1/1
  In1/1 -> Demux/1
  Demux/2 -> Mux/2
  Demux/3 -> Mux/3, Out2/1
  Demux/1 -> Mux/1
  Demux/5 -> Mux/5, Mux1/2

== system Perfect_Lineaer/Skid to turn (Lateral Dynamics)2/Subsystem3/selector ==
  note: Outer loop
  In1 : Inport
  Demux : Demux  Outputs=9
  Demux1 : Demux  Outputs=3
  MATLAB Function : MATLAB Function  TreatAsAtomicUnit=on
  Mux : Mux  Inputs=8
  Mux1 : Mux  Inputs=3
  Scope : Scope
  Terminator : Terminator
  Terminator1 : Terminator
  Terminator2 : Terminator
  Out1 : Outport
  Out2 : Outport  Port=2
  wires:
  Mux1/1 -> Scope/1
  Demux/9 -> Mux/8
  Demux/8 -> Out1/1
  Mux/1 -> Terminator/1
  Demux/7 -> Mux/7
  Demux/6 -> Mux/6, Mux1/3
  Demux/4 -> MATLAB Function/1(phi), Mux/4, Mux1/1
  In1/1 -> Demux/1
  Demux/2 -> MATLAB Function/5(R), Mux/2
  Demux/3 -> Mux/3
  Demux/1 -> MATLAB Function/4(Q), MATLAB Function/3(P), Mux/1
  Demux/5 -> MATLAB Function/2(theta), Mux/5, Mux1/2
  MATLAB Function/1(euler_dot) -> Demux1/1
  Demux1/2 -> Out2/1
  Demux1/1 -> Terminator1/1
  Demux1/3 -> Terminator2/1

== system Perfect_Lineaer/Skid to turn (Lateral Dynamics)2/Subsystem4/selector ==
  note: Outer loop
  In1 : Inport
  Demux : Demux  Outputs=9
  Mux : Mux  Inputs=8
  Mux1 : Mux  Inputs=3
  Scope : Scope
  Terminator : Terminator
  Out1 : Outport
  Out2 : Outport  Port=2
  wires:
  Mux1/1 -> Scope/1
  Demux/9 -> Mux/8
  Demux/8 -> Out1/1
  Mux/1 -> Terminator/1
  Demux/7 -> Mux/7
  Demux/6 -> Mux/6, Mux1/3
  Demux/4 -> Mux/4, Mux1/1
  In1/1 -> Demux/1
  Demux/2 -> Mux/2
  Demux/3 -> Mux/3
  Demux/1 -> Mux/1
  Demux/5 -> Mux/5, Out2/1

== system Perfect_Lineaer/Skid to turn (Lateral Dynamics)2/Subsystem5/selector ==
  note: Outer loop
  In1 : Inport
  Demux : Demux  Outputs=9
  Demux1 : Demux  Outputs=3
  MATLAB Function : MATLAB Function  TreatAsAtomicUnit=on
  Mux : Mux  Inputs=8
  Mux1 : Mux  Inputs=3
  Scope : Scope
  Terminator : Terminator
  Terminator1 : Terminator
  Out1 : Outport
  Out2 : Outport  Port=2
  Out3 : Outport  Port=3
  wires:
  MATLAB Function/1(euler_dot) -> Demux1/1
  Demux1/1 -> Terminator1/1
  In1/1 -> Demux/1
  Demux/9 -> Mux/8
  Demux/5 -> MATLAB Function/2(theta), Mux/5, Mux1/2
  Demux/2 -> MATLAB Function/5(R), Mux/2
  Demux/6 -> Mux/6, Mux1/3
  Demux/1 -> MATLAB Function/4(Q), MATLAB Function/3(P), Mux/1
  Demux/3 -> Mux/3
  Mux/1 -> Terminator/1
  Demux/7 -> Mux/7
  Demux/4 -> MATLAB Function/1(phi), Mux/4, Mux1/1
  Demux1/2 -> Out2/1
  Demux/8 -> Out1/1
  Mux1/1 -> Scope/1
  Demux1/3 -> Out3/1

== system Perfect_Lineaer/Skid to turn (Lateral Dynamics)2/Subsystem6/selector ==
  note: Outer loop
  In1 : Inport
  Demux : Demux  Outputs=9
  Mux : Mux  Inputs=8
  Mux1 : Mux  Inputs=3
  Scope : Scope
  Terminator : Terminator
  Out1 : Outport
  Out2 : Outport  Port=2
  wires:
  Mux1/1 -> Scope/1
  Demux/9 -> Mux/8
  Demux/8 -> Out1/1
  Mux/1 -> Terminator/1
  Demux/7 -> Mux/7
  Demux/6 -> Mux/6, Mux1/3
  Demux/4 -> Mux/4, Mux1/1
  In1/1 -> Demux/1
  Demux/2 -> Mux/2
  Demux/3 -> Mux/3, Out2/1
  Demux/1 -> Mux/1
  Demux/5 -> Mux/5, Mux1/2

== system Perfect_Lineaer/Skid to turn (Lateral Dynamics)2/Subsystem7/selector ==
  note: Outer loop
  In1 : Inport
  Demux : Demux  Outputs=9
  Demux1 : Demux  Outputs=3
  MATLAB Function : MATLAB Function  TreatAsAtomicUnit=on
  Mux : Mux  Inputs=8
  Mux1 : Mux  Inputs=3
  Scope : Scope
  Terminator : Terminator
  Terminator1 : Terminator
  Terminator2 : Terminator
  Out1 : Outport
  Out2 : Outport  Port=2
  wires:
  MATLAB Function/1(euler_dot) -> Demux1/1
  Demux1/3 -> Terminator2/1
  In1/1 -> Demux/1
  Demux/9 -> Mux/8
  Demux/5 -> MATLAB Function/2(theta), Mux/5, Mux1/2
  Demux/2 -> MATLAB Function/5(R), Mux/2
  Demux/6 -> Mux/6, Mux1/3
  Demux/1 -> MATLAB Function/4(Q), MATLAB Function/3(P), Mux/1
  Demux/3 -> Mux/3
  Mux/1 -> Terminator/1
  Demux/7 -> Mux/7
  Demux/4 -> MATLAB Function/1(phi), Mux/4, Mux1/1
  Demux/8 -> Out1/1
  Mux1/1 -> Scope/1
  Demux1/2 -> Terminator1/1
  Demux1/1 -> Out2/1

== system Perfect_Lineaer/Skid to turn (Lateral Dynamics)2/Subsystem8/selector ==
  note: Outer loop
  In1 : Inport
  Demux : Demux  Outputs=9
  Demux1 : Demux  Outputs=3
  MATLAB Function : MATLAB Function  TreatAsAtomicUnit=on
  Mux : Mux  Inputs=8
  Mux1 : Mux  Inputs=3
  Scope : Scope
  Terminator : Terminator
  Terminator1 : Terminator
  Terminator2 : Terminator
  Out1 : Outport
  Out2 : Outport  Port=2
  wires:
  Demux1/2 -> Terminator1/1
  Demux/7 -> Mux/7
  Demux/3 -> Mux/3
  Mux/1 -> Terminator/1
  Demux/2 -> MATLAB Function/5(R), Mux/2
  In1/1 -> Demux/1
  Demux/5 -> MATLAB Function/2(theta), Mux/5, Mux1/2
  Demux/9 -> Mux/8
  Demux/6 -> Mux/6, Mux1/3
  Demux1/3 -> Terminator2/1
  MATLAB Function/1(euler_dot) -> Demux1/1
  Mux1/1 -> Scope/1
  Demux/4 -> MATLAB Function/1(phi), Mux/4, Mux1/1
  Demux/1 -> MATLAB Function/4(Q), MATLAB Function/3(P), Mux/1
  Demux1/1 -> Out2/1
  Demux/8 -> Out1/1

== system Perfect_Lineaer/Skid to turn (Lateral Dynamics)2/Subsystem9/selector ==
  note: Outer loop
  In1 : Inport
  Demux : Demux  Outputs=9
  Demux1 : Demux  Outputs=3
  MATLAB Function : MATLAB Function  TreatAsAtomicUnit=on
  Mux : Mux  Inputs=8
  Mux1 : Mux  Inputs=3
  Scope : Scope
  Terminator : Terminator
  Terminator1 : Terminator
  Terminator2 : Terminator
  Out1 : Outport
  Out2 : Outport  Port=2
  wires:
  Demux1/2 -> Terminator1/1
  Demux/7 -> Mux/7
  Demux/3 -> Mux/3
  Mux/1 -> Terminator/1
  Demux/2 -> MATLAB Function/5(R), Mux/2
  In1/1 -> Demux/1
  Demux/5 -> MATLAB Function/2(theta), Mux/5, Mux1/2
  Demux/9 -> Mux/8
  Demux/6 -> Mux/6, Mux1/3
  Demux1/3 -> Terminator2/1
  MATLAB Function/1(euler_dot) -> Demux1/1
  Mux1/1 -> Scope/1
  Demux/4 -> MATLAB Function/1(phi), Mux/4, Mux1/1
  Demux/1 -> MATLAB Function/4(Q), MATLAB Function/3(P), Mux/1
  Demux1/1 -> Out2/1
  Demux/8 -> Out1/1

== system Perfect_Lineaer/Subsystem1/Subsystem/selector ==
  note: Outer loop
  In1 : Inport
  Demux : Demux  Outputs=9
  Mux : Mux  Inputs=8
  Mux1 : Mux  Inputs=3
  Scope : Scope
  Terminator : Terminator
  Out1 : Outport
  Out2 : Outport  Port=2
  wires:
  Demux/5 -> Mux1/2, Mux/5
  Demux/1 -> Mux/1
  Demux/3 -> Out2/1, Mux/3
  Demux/2 -> Mux/2
  In1/1 -> Demux/1
  Demux/4 -> Mux1/1, Mux/4
  Demux/6 -> Mux1/3, Mux/6
  Demux/7 -> Mux/7
  Mux/1 -> Terminator/1
  Demux/8 -> Out1/1
  Demux/9 -> Mux/8
  Mux1/1 -> Scope/1

== system Perfect_Lineaer/Subsystem1/Subsystem1/selector ==
  note: Outer loop
  In1 : Inport
  Demux : Demux  Outputs=9
  Mux : Mux  Inputs=8
  Mux1 : Mux  Inputs=3
  Scope : Scope
  Terminator : Terminator
  Out1 : Outport
  Out2 : Outport  Port=2
  wires:
  Demux/5 -> Mux1/2, Mux/5
  Demux/1 -> Mux/1
  Demux/3 -> Mux/3
  Demux/2 -> Out2/1, Mux/2
  In1/1 -> Demux/1
  Demux/4 -> Mux1/1, Mux/4
  Demux/6 -> Mux1/3, Mux/6
  Demux/7 -> Mux/7
  Mux/1 -> Terminator/1
  Demux/8 -> Out1/1
  Demux/9 -> Mux/8
  Mux1/1 -> Scope/1

== system Perfect_Lineaer/Subsystem1/Subsystem5/selector ==
  note: Outer loop
  In1 : Inport
  Demux : Demux  Outputs=9
  Mux : Mux  Inputs=8
  Mux1 : Mux  Inputs=3
  Scope : Scope
  Terminator : Terminator
  Out1 : Outport
  yaw : Outport  Port=2
  pitch : Outport  Port=3
  wires:
  Demux/5 -> Mux1/2, Mux/5
  Demux/1 -> Mux/1
  Demux/3 -> yaw/1, Mux/3
  Demux/2 -> pitch/1, Mux/2
  In1/1 -> Demux/1
  Demux/4 -> Mux1/1, Mux/4
  Demux/6 -> Mux1/3, Mux/6
  Demux/7 -> Mux/7
  Mux/1 -> Terminator/1
  Demux/8 -> Out1/1
  Demux/9 -> Mux/8
  Mux1/1 -> Scope/1

== system Perfect_Lineaer/Washout/Subsystem/selector ==
  note: Outer loop
  In1 : Inport
  Demux : Demux  Outputs=9
  Demux1 : Demux  Outputs=3
  MATLAB Function : MATLAB Function  TreatAsAtomicUnit=on
  Mux : Mux  Inputs=8
  Mux1 : Mux  Inputs=3
  Scope : Scope
  Terminator : Terminator
  Terminator1 : Terminator
  Terminator2 : Terminator
  Out1 : Outport
  Out2 : Outport  Port=2
  Out3 : Outport  Port=3
  wires:
  MATLAB Function/1(euler_dot) -> Demux1/1
  Demux1/1 -> Terminator1/1
  In1/1 -> Demux/1
  Demux/9 -> Mux/8
  Demux/5 -> MATLAB Function/2(theta), Mux/5, Mux1/2
  Demux/2 -> MATLAB Function/5(R), Mux/2
  Demux/6 -> Mux/6, Out3/1, Mux1/3
  Demux/1 -> MATLAB Function/4(Q), MATLAB Function/3(P), Mux/1
  Demux/3 -> Mux/3
  Mux/1 -> Terminator/1
  Demux/7 -> Mux/7
  Demux/4 -> MATLAB Function/1(phi), Mux/4, Mux1/1
  Demux/8 -> Out1/1
  Mux1/1 -> Scope/1
  Demux1/3 -> Out2/1
  Demux1/2 -> Terminator2/1

== system Perfect_Lineaer/Washout/Subsystem1/selector ==
  note: Outer loop
  In1 : Inport
  Demux : Demux  Outputs=9
  Demux1 : Demux  Outputs=3
  MATLAB Function : MATLAB Function  TreatAsAtomicUnit=on
  Mux : Mux  Inputs=8
  Mux1 : Mux  Inputs=3
  Scope : Scope
  Terminator : Terminator
  Terminator1 : Terminator
  Terminator2 : Terminator
  Out1 : Outport
  Out2 : Outport  Port=2
  Out3 : Outport  Port=3
  wires:
  MATLAB Function/1(euler_dot) -> Demux1/1
  Demux1/1 -> Terminator1/1
  In1/1 -> Demux/1
  Demux/9 -> Mux/8
  Demux/5 -> MATLAB Function/2(theta), Mux/5, Mux1/2
  Demux/2 -> MATLAB Function/5(R), Mux/2
  Demux/1 -> MATLAB Function/4(Q), MATLAB Function/3(P), Mux/1
  Demux/3 -> Mux/3
  Mux/1 -> Terminator/1
  Demux/7 -> Mux/7
  Demux/4 -> MATLAB Function/1(phi), Mux/4, Mux1/1
  Demux/8 -> Out1/1
  Mux1/1 -> Scope/1
  Demux1/3 -> Out2/1
  Demux1/2 -> Terminator2/1
  Demux/6 -> Mux/6, Out3/1, Mux1/3

== system Perfect_Lineaer/Washout/Subsystem2/selector ==
  note: Outer loop
  In1 : Inport
  Demux : Demux  Outputs=9
  Mux : Mux  Inputs=8
  Mux1 : Mux  Inputs=3
  Scope : Scope
  Terminator : Terminator
  Out1 : Outport
  Out2 : Outport  Port=2
  wires:
  Demux/5 -> Mux1/2, Mux/5
  Demux/1 -> Mux/1
  Demux/3 -> Out2/1, Mux/3
  Demux/2 -> Mux/2
  In1/1 -> Demux/1
  Demux/4 -> Mux1/1, Mux/4
  Demux/6 -> Mux1/3, Mux/6
  Demux/7 -> Mux/7
  Mux/1 -> Terminator/1
  Demux/8 -> Out1/1
  Demux/9 -> Mux/8
  Mux1/1 -> Scope/1

== system Perfect_Lineaer/Washout/Subsystem3/selector ==
  note: Outer loop
  In1 : Inport
  Demux : Demux  Outputs=9
  Mux : Mux  Inputs=8
  Mux1 : Mux  Inputs=3
  Scope : Scope
  Terminator : Terminator
  Out1 : Outport
  Out2 : Outport  Port=2
  wires:
  Demux/5 -> Mux1/2, Mux/5
  Demux/1 -> Mux/1
  Demux/3 -> Out2/1, Mux/3
  Demux/2 -> Mux/2
  In1/1 -> Demux/1
  Demux/4 -> Mux1/1, Mux/4
  Demux/6 -> Mux1/3, Mux/6
  Demux/7 -> Mux/7
  Mux/1 -> Terminator/1
  Demux/8 -> Out1/1
  Demux/9 -> Mux/8
  Mux1/1 -> Scope/1

== system Perfect_Lineaer/Washout/Subsystem4/selector ==
  note: Outer loop
  In1 : Inport
  Demux : Demux  Outputs=9
  Mux : Mux  Inputs=8
  Mux1 : Mux  Inputs=3
  Scope : Scope
  Terminator : Terminator
  Out1 : Outport
  Out2 : Outport  Port=2
  wires:
  Demux/5 -> Mux1/2, Mux/5
  Demux/1 -> Mux/1
  Demux/3 -> Out2/1, Mux/3
  Demux/2 -> Mux/2
  In1/1 -> Demux/1
  Demux/4 -> Mux1/1, Mux/4
  Demux/6 -> Mux1/3, Mux/6
  Demux/7 -> Mux/7
  Mux/1 -> Terminator/1
  Demux/8 -> Out1/1
  Demux/9 -> Mux/8
  Mux1/1 -> Scope/1

== system Perfect_Lineaer/All together/Subsystem1/new tran kine sph/X_EE 2 P_EE ==
  X_E_E_BE : Inport
  Rearth : Inport  Port=2
  Add : Sum  Inputs=+-
  Atan1 : Trigonometry  Operator=asin
  Atan2 : Trigonometry  Operator=atan2
  Demux : Demux  Outputs=3
  Divide : Product  Inputs=*/
  Dot Product1 : DotProduct  InputSameDT=on  OutDataTypeStr=Inherit: Inherit via internal rule
  Mux1 : Mux  Inputs=3
  Signed Sqrt1 : Sqrt  SaturateOnIntegerOverflow=on
  P_E_E_BE : Outport
  wires:
  X_E_E_BE/1 -> Dot Product1/2, Dot Product1/1, Demux/1
  Demux/1 -> Atan2/2
  Demux/2 -> Atan2/1
  Atan2/1 -> Mux1/2
  Dot Product1/1 -> Signed Sqrt1/1
  Signed Sqrt1/1 -> Add/1
  Rearth/1 -> Divide/2, Add/2
  Add/1 -> Mux1/3
  Mux1/1 -> P_E_E_BE/1
  Demux/3 -> Divide/1
  Divide/1 -> Atan1/1
  Atan1/1 -> Mux1/1

== system Perfect_Lineaer/All together/Subsystem1/new tran kine sph/X_EE 2 P_EE1 ==
  X_E_E_BE : Inport
  Rearth : Inport  Port=2
  Add : Sum  Inputs=+-
  Atan1 : Trigonometry  Operator=atan2
  Atan2 : Trigonometry  Operator=atan2
  Demux : Demux  Outputs=3
  Dot Product : DotProduct  InputSameDT=on  OutDataTypeStr=Inherit: Inherit via internal rule
  Dot Product1 : DotProduct  InputSameDT=on  OutDataTypeStr=Inherit: Inherit via internal rule
  Mux : Mux  Inputs=2
  Mux1 : Mux  Inputs=3
  Signed Sqrt : Sqrt  SaturateOnIntegerOverflow=on
  Signed Sqrt1 : Sqrt  SaturateOnIntegerOverflow=on
  P_E_E_BE : Outport
  wires:
  X_E_E_BE/1 -> Dot Product1/2, Dot Product1/1, Demux/1
  Demux/1 -> Mux/1, Atan2/2
  Demux/2 -> Atan2/1, Mux/2
  Mux/1 -> Dot Product/2, Dot Product/1
  Dot Product/1 -> Signed Sqrt/1
  Signed Sqrt/1 -> Atan1/2
  Demux/3 -> Atan1/1
  Atan2/1 -> Mux1/2
  Atan1/1 -> Mux1/1
  Dot Product1/1 -> Signed Sqrt1/1
  Signed Sqrt1/1 -> Add/1
  Rearth/1 -> Add/2
  Add/1 -> Mux1/3
  Mux1/1 -> P_E_E_BE/1

== system Perfect_Lineaer/All together/Subsystem1/new tran kine sph/p2Cne ==
  p_E_E_BE : Inport
  Constant : Constant  Value=[0 0 1; 0 1 0;-1 0 0]
  Demux : Demux  Outputs=3
  LAT DCM : MATLAB Function  TreatAsAtomicUnit=on
  LON DCM : MATLAB Function  TreatAsAtomicUnit=on
  Matrix Multiply : Product  Multiplication=Matrix(*)
  Matrix Multiply1 : Product  Multiplication=Matrix(*)
  Scope1 : Scope
  Terminator : Terminator
  C-NE : Outport
  wires:
  p_E_E_BE/1 -> Demux/1
  Demux/3 -> Terminator/1
  Demux/2 -> LON DCM/1(u)
  Demux/1 -> LAT DCM/1(u)
  LAT DCM/1(y) -> Matrix Multiply/1
  LON DCM/1(y) -> Matrix Multiply/2
  Matrix Multiply/1 -> Matrix Multiply1/1
  Constant/1 -> Matrix Multiply1/2
  Matrix Multiply1/1 -> Scope1/1, C-NE/1

== matlab function Perfect_Lineaer/Skid to turn (Lateral Dynamics)2/Subsystem1/selector/MATLAB Function ==
  data: phi input; euler_dot output; theta input; P input; Q input; R input
function euler_dot= fcn(phi,theta,P,Q,R)
A=[P;Q;R];
%psi=theta(3); %not needed for Euler Rotational Kinematics Matrix
matrix=[1,tan(theta)*sin(phi),tan(theta)*cos(phi); 0,cos(phi),-sin(phi);0,sin(phi)/cos(theta),cos(phi)/cos(theta)];
euler_dot=matrix*A;

== matlab function Perfect_Lineaer/Skid to turn (Lateral Dynamics)2/Subsystem3/selector/MATLAB Function ==
  data: phi input; euler_dot output; theta input; P input; Q input; R input
function euler_dot= fcn(phi,theta,P,Q,R)
A=[P;Q;R];
%psi=theta(3); %not needed for Euler Rotational Kinematics Matrix
matrix=[1,tan(theta)*sin(phi),tan(theta)*cos(phi); 0,cos(phi),-sin(phi);0,sin(phi)/cos(theta),cos(phi)/cos(theta)];
euler_dot=matrix*A;

== matlab function Perfect_Lineaer/Skid to turn (Lateral Dynamics)2/Subsystem/selector/MATLAB Function ==
  data: phi input; euler_dot output; theta input; P input; Q input; R input
function euler_dot= fcn(phi,theta,P,Q,R)
A=[P;Q;R];
%psi=theta(3); %not needed for Euler Rotational Kinematics Matrix
matrix=[1,tan(theta)*sin(phi),tan(theta)*cos(phi); 0,cos(phi),-sin(phi);0,sin(phi)/cos(theta),cos(phi)/cos(theta)];
euler_dot=matrix*A;

== matlab function Perfect_Lineaer/Skid to turn (Lateral Dynamics)2/Subsystem5/selector/MATLAB Function ==
  data: phi input; euler_dot output; theta input; P input; Q input; R input
function euler_dot= fcn(phi,theta,P,Q,R)
A=[P;Q;R];
%psi=theta(3); %not needed for Euler Rotational Kinematics Matrix
matrix=[1,tan(theta)*sin(phi),tan(theta)*cos(phi); 0,cos(phi),-sin(phi);0,sin(phi)/cos(theta),cos(phi)/cos(theta)];
euler_dot=matrix*A;

== matlab function Perfect_Lineaer/Skid to turn (Lateral Dynamics)2/Subsystem7/selector/MATLAB Function ==
  data: phi input; euler_dot output; theta input; P input; Q input; R input
function euler_dot= fcn(phi,theta,P,Q,R)
A=[P;Q;R];
%psi=theta(3); %not needed for Euler Rotational Kinematics Matrix
matrix=[1,tan(theta)*sin(phi),tan(theta)*cos(phi); 0,cos(phi),-sin(phi);0,sin(phi)/cos(theta),cos(phi)/cos(theta)];
euler_dot=matrix*A;

== matlab function Perfect_Lineaer/Skid to turn (Lateral Dynamics)2/Subsystem8/selector/MATLAB Function ==
  data: phi input; euler_dot output; theta input; P input; Q input; R input
function euler_dot= fcn(phi,theta,P,Q,R)
A=[P;Q;R];
%psi=theta(3); %not needed for Euler Rotational Kinematics Matrix
matrix=[1,tan(theta)*sin(phi),tan(theta)*cos(phi); 0,cos(phi),-sin(phi);0,sin(phi)/cos(theta),cos(phi)/cos(theta)];
euler_dot=matrix*A;

== matlab function Perfect_Lineaer/Skid to turn (Lateral Dynamics)2/Subsystem9/selector/MATLAB Function ==
  data: phi input; euler_dot output; theta input; P input; Q input; R input
function euler_dot= fcn(phi,theta,P,Q,R)
A=[P;Q;R];
%psi=theta(3); %not needed for Euler Rotational Kinematics Matrix
matrix=[1,tan(theta)*sin(phi),tan(theta)*cos(phi); 0,cos(phi),-sin(phi);0,sin(phi)/cos(theta),cos(phi)/cos(theta)];
euler_dot=matrix*A;

== matlab function Perfect_Lineaer/Command size/Subsystem3/selector/MATLAB Function ==
  data: phi input; euler_dot output; theta input; P input; Q input; R input
function euler_dot= fcn(phi,theta,P,Q,R)
A=[P;Q;R];
%psi=theta(3); %not needed for Euler Rotational Kinematics Matrix
matrix=[1,tan(theta)*sin(phi),tan(theta)*cos(phi); 0,cos(phi),-sin(phi);0,sin(phi)/cos(theta),cos(phi)/cos(theta)];
euler_dot=matrix*A;

== matlab function Perfect_Lineaer/Command size/Subsystem1/selector/MATLAB Function ==
  data: phi input; euler_dot output; theta input; P input; Q input; R input
function euler_dot= fcn(phi,theta,P,Q,R)
A=[P;Q;R];
%psi=theta(3); %not needed for Euler Rotational Kinematics Matrix
matrix=[1,tan(theta)*sin(phi),tan(theta)*cos(phi); 0,cos(phi),-sin(phi);0,sin(phi)/cos(theta),cos(phi)/cos(theta)];
euler_dot=matrix*A;

== matlab function Perfect_Lineaer/Command size/Subsystem/selector/MATLAB Function ==
  data: phi input; euler_dot output; theta input; P input; Q input; R input
function euler_dot= fcn(phi,theta,P,Q,R)
A=[P;Q;R];
%psi=theta(3); %not needed for Euler Rotational Kinematics Matrix
matrix=[1,tan(theta)*sin(phi),tan(theta)*cos(phi); 0,cos(phi),-sin(phi);0,sin(phi)/cos(theta),cos(phi)/cos(theta)];
euler_dot=matrix*A;

== matlab function Perfect_Lineaer/Command size/Subsystem2/selector/MATLAB Function ==
  data: phi input; euler_dot output; theta input; P input; Q input; R input
function euler_dot= fcn(phi,theta,P,Q,R)
A=[P;Q;R];
%psi=theta(3); %not needed for Euler Rotational Kinematics Matrix
matrix=[1,tan(theta)*sin(phi),tan(theta)*cos(phi); 0,cos(phi),-sin(phi);0,sin(phi)/cos(theta),cos(phi)/cos(theta)];
euler_dot=matrix*A;

== matlab function Perfect_Lineaer/Command size/Subsystem9/selector/MATLAB Function ==
  data: phi input; euler_dot output; theta input; P input; Q input; R input
function euler_dot= fcn(phi,theta,P,Q,R)
A=[P;Q;R];
%psi=theta(3); %not needed for Euler Rotational Kinematics Matrix
matrix=[1,tan(theta)*sin(phi),tan(theta)*cos(phi); 0,cos(phi),-sin(phi);0,sin(phi)/cos(theta),cos(phi)/cos(theta)];
euler_dot=matrix*A;

== matlab function Perfect_Lineaer/Command size/Subsystem4/selector/MATLAB Function ==
  data: phi input; euler_dot output; theta input; P input; Q input; R input
function euler_dot= fcn(phi,theta,P,Q,R)
A=[P;Q;R];
%psi=theta(3); %not needed for Euler Rotational Kinematics Matrix
matrix=[1,tan(theta)*sin(phi),tan(theta)*cos(phi); 0,cos(phi),-sin(phi);0,sin(phi)/cos(theta),cos(phi)/cos(theta)];
euler_dot=matrix*A;

== matlab function Perfect_Lineaer/Pilot command(STT)/Subsystem/selector/MATLAB Function ==
  data: phi input; euler_dot output; theta input; P input; Q input; R input
function euler_dot= fcn(phi,theta,P,Q,R)
A=[P;Q;R];
%psi=theta(3); %not needed for Euler Rotational Kinematics Matrix
matrix=[1,tan(theta)*sin(phi),tan(theta)*cos(phi); 0,cos(phi),-sin(phi);0,sin(phi)/cos(theta),cos(phi)/cos(theta)];
euler_dot=matrix*A;

== matlab function Perfect_Lineaer/Pilot command(STT)/Subsystem1/selector/MATLAB Function ==
  data: phi input; euler_dot output; theta input; P input; Q input; R input
function euler_dot= fcn(phi,theta,P,Q,R)
A=[P;Q;R];
%psi=theta(3); %not needed for Euler Rotational Kinematics Matrix
matrix=[1,tan(theta)*sin(phi),tan(theta)*cos(phi); 0,cos(phi),-sin(phi);0,sin(phi)/cos(theta),cos(phi)/cos(theta)];
euler_dot=matrix*A;

== matlab function Perfect_Lineaer/Pilot command(STT)/Subsystem5/selector/MATLAB Function ==
  data: phi input; euler_dot output; theta input; P input; Q input; R input
function euler_dot= fcn(phi,theta,P,Q,R)
A=[P;Q;R];
%psi=theta(3); %not needed for Euler Rotational Kinematics Matrix
matrix=[1,tan(theta)*sin(phi),tan(theta)*cos(phi); 0,cos(phi),-sin(phi);0,sin(phi)/cos(theta),cos(phi)/cos(theta)];
euler_dot=matrix*A;

== matlab function Perfect_Lineaer/Decoupled/Subsystem5/selector/MATLAB Function ==
  data: phi input; euler_dot output; theta input; P input; Q input; R input
function euler_dot= fcn(phi,theta,P,Q,R)
A=[P;Q;R];
%psi=theta(3); %not needed for Euler Rotational Kinematics Matrix
matrix=[1,tan(theta)*sin(phi),tan(theta)*cos(phi); 0,cos(phi),-sin(phi);0,sin(phi)/cos(theta),cos(phi)/cos(theta)];
euler_dot=matrix*A;
